simulink model "dcmotorspeedcontroll"  (Simulink 8.7)
settings: Solver=FixedStepDiscrete  StartTime=0.0  StopTime=10  FixedStep=ts  RelTol=1e-3
undefined symbols (not defined in the file or in its folder): ts
libraries: powerlib x4
settings Model: Creator=Aditya  LastModifiedBy=Aditya
settings DataIOCC: LimitDataPoints=off  SaveFormat=Dataset
settings DebuggingCC: UnderspecifiedInitializationDetection=Simplified  MergeDetectMultiDrivingBlocksExec=error
settings HardwareCC: ProdBitPerPointer=64  ProdLargestAtomicFloat=Float  ProdIntDivRoundTo=Zero  ProdEndianess=LittleEndian  ProdWordSize=64  ProdHWDeviceType=Intel->x86-64 (Windows64)
settings ModelReferenceCC: PropagateSignalLabelsOutOfModel=on
settings ConfigComp: CovModelRefEnable=off

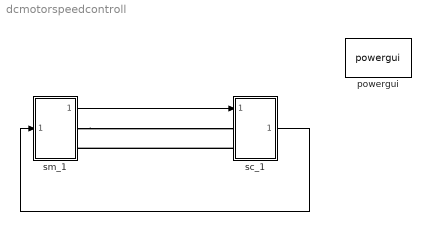
== system dcmotorspeedcontroll ==
  powergui : powerlib/powergui  Priority=1  SimulationMode=Discrete  SolverType=Tustin/Backward Euler (TBE)  SampleTime=ts  frequency=60  SPID=off  DisableSnubberDevices=off  DisableRonSwitches=off  DisableVfSwitches=off  SwTol=0  DisplayEquations=off  Interpol=off  ExternalGateDelay=off  methode=off  Ts=10  FunctionMessages=off  echomessages=off  HookPort=off  EnableUseOfTLC=off  x0status=blocks  frequencyindice=0  Pbase=100e6  ErrMax=1e-4  Iterations=50  UnitsV=kV  UnitsW=MW  buscounter=0  RestoreLinks=warning  ResistiveCurrentMeasurement=off  Frange=[0:2:500]  Ylog=off  Xlog=on  ShowGrid=off  save=off  variable=ZData  structure=0  ZoomFFT=off  StartTime=0.0  cycles=1  DisplayStyle=1  fundamental=60  FreqAxis=off  MaxFrequency=1000  frequencyindicesteady=1  RmsSteady=1  display=off
  sc_1 : Subsystem
  sm_1 : Subsystem
  wires:
  sm_1/1(Out1) -> sc_1/1(In1)
  sc_1/1(Out1) -> sm_1/1(In1)
  connections:
  sm_1/RConn1 -- sc_1/LConn1
  sc_1/LConn2 -- sm_1/RConn2

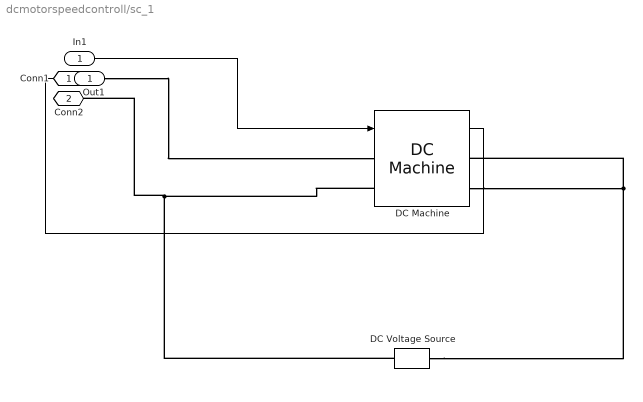
== system dcmotorspeedcontroll/sc_1 ==
  In1 : Inport
  DC Machine : powerlib/Machines/DC Machine  PresetModel=No  MechanicalLoad=Torque TL  FieldType=Wound  ShowDetailedParameters=on  MeasurementBus=off  RLa="[ 0.6  0.012]"  RLf="[ 240  120]"  Laf=1.8  MachineConstant=Torque constant (N.m/A)  Ke=1.8  Kt=1.8  J=1  Bm=0  Tf=0  w0=1  Ifinit=1  TsPowergui=0  TsBlock=-1
  DC Voltage Source : powerlib/Electrical Sources/DC Voltage Source  Amplitude=100  Measurements=None
  Conn1 : PMIOPort  Port=1  Side=Left
  Conn2 : PMIOPort  Port=2  Side=Left
  Out1 : Outport
  wires:
  In1/1 -> DC Machine/1
  DC Machine/1 -> Out1/1
  connections:
  DC Voltage Source/LConn1 -- DC Machine/RConn2 -- DC Machine/RConn1
  DC Voltage Source/RConn1 -- Conn2/RConn1 -- DC Machine/LConn2
  Conn1/RConn1 -- DC Machine/LConn1

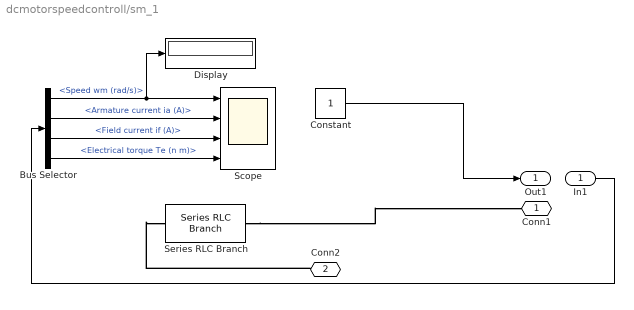
== system dcmotorspeedcontroll/sm_1 ==
  In1 : Inport
  Bus Selector : BusSelector  OutputSignals=Speed wm (rad/s),Armature current ia (A),Field current if (A),Electrical torque Te (n m)
  Constant : Constant
  Display : Display
  Scope : Scope  NumInputPorts=4
  Series RLC Branch : powerlib/Elements/Series RLC Branch  LConnTagsString=__new0  RConnTagsString=__new0  BranchType=R  Resistance=5  Inductance=1e-3  SetiL0=off  InitialCurrent=0  Capacitance=1e-6  Setx0=off  InitialVoltage=0  Measurements=None
  Conn1 : PMIOPort  Port=1  Side=Right
  Conn2 : PMIOPort  Port=2  Side=Right
  Out1 : Outport
  wires:
  Constant/1 -> Out1/1
  In1/1 -> Bus Selector/1
  Bus Selector/3 -> Scope/3  "<Field current if (A)>"
  Bus Selector/2 -> Scope/2  "<Armature current ia (A)>"
  Bus Selector/4 -> Scope/4  "<Electrical torque Te (n m)>"
  Bus Selector/1 -> Display/1, Scope/1  "<Speed wm (rad/s)>"
  connections:
  Series RLC Branch/RConn1 -- Conn1/RConn1
  Conn2/RConn1 -- Series RLC Branch/LConn1
